simulink subsystem "Diagnostic_Reporter"  (R2023a)
settings: Solver=VariableStepAuto  StartTime=0.0  StopTime=10.0  RelTol=1e-3
undefined symbols (not defined in the file or in its folder): header, key, key_SL_Info, level, message, message_SL_Info, name, name_SL_Info, status, status_SL_Info, value, value_SL_Info, values, values_SL_Info
libraries: ros2lib x13
settings Model: Creator=hollis  LastModifiedBy=john

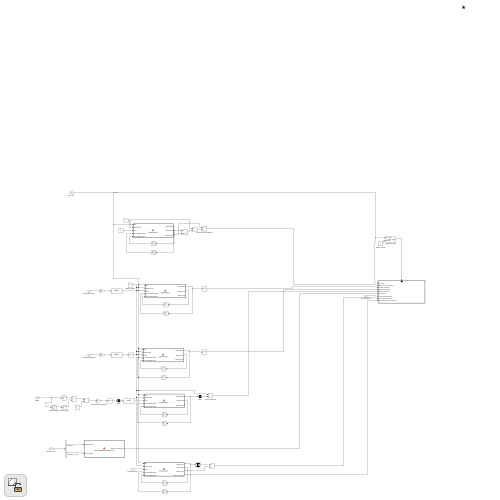
[thumbnail: Simulink's stored preview of the top-level diagram]
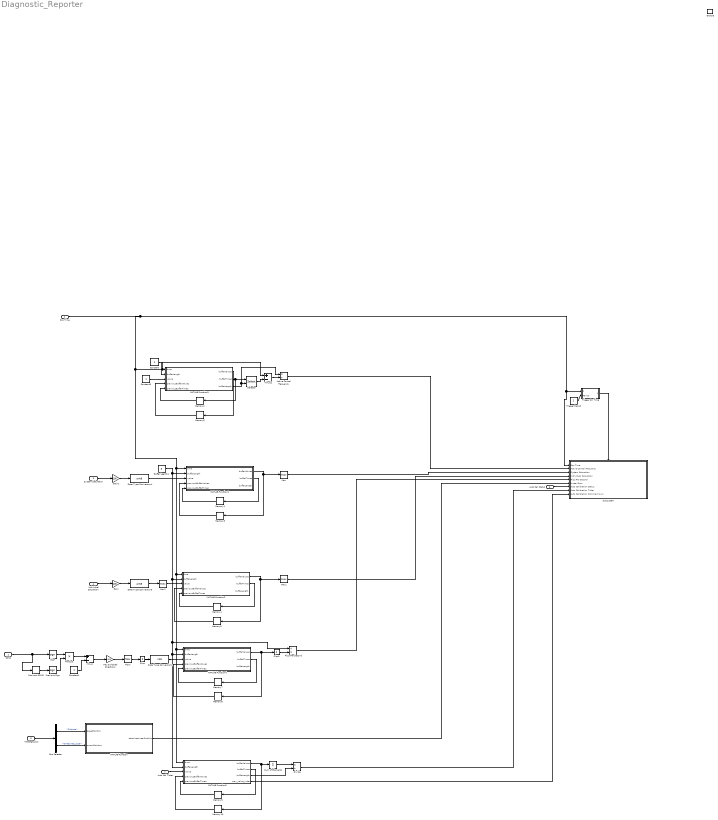
== system Diagnostic_Reporter ==
  Ros Time : Inport
  RPMs : Inport  Port=2
  System Saturation : Inport  Port=3
  Individual Saturation : Inport  Port=4
  message_bus : Inport  Port=5
  Auto Cal Status : Inport  Port=6
  Auto Cal Ticker : Inport  Port=7
  Enable : EnablePort
  Active Control Frequency : Product  Inputs=*/
  Buffer Legnth1 : Constant  Value=3
  Bus Selector : BusSelector  OutputSignals=current_state.DApose,desired_pose.DAdesired_pose
  Constant : Constant
  Constant1 : Constant
  Constant3 : Constant  OutDataTypeStr=single
  Data Type Conversion1 : DataTypeConversion  OutDataTypeStr=int8  SaturateOnIntegerOverflow=off  RndMeth=Floor
  Data Type Conversion3 : DataTypeConversion  OutDataTypeStr=uint8  SaturateOnIntegerOverflow=off  RndMeth=Floor
  Data Type Conversion4 : DataTypeConversion  OutDataTypeStr=uint8  SaturateOnIntegerOverflow=off  RndMeth=Floor
  Divide : Product  Inputs=*/
  Flips : Sum  Inputs=+
  Flips Per Second : Product  Inputs=/*
  Flips1 : Sum  Inputs=+
  Floor : Rounding
  Gain : Gain  Gain=100
  Gain1 : Gain  Gain=100
  Has Switched Directions : Gain  Gain=-1/2
  MATLAB Function : MATLAB Function  TreatAsAtomicUnit=on
  MATLAB Function1 : MATLAB Function  TreatAsAtomicUnit=on
  MATLAB Function2 : MATLAB Function  TreatAsAtomicUnit=on
  MATLAB Function3 : MATLAB Function  TreatAsAtomicUnit=on
  MATLAB Function4 : MATLAB Function  TreatAsAtomicUnit=on
  MATLAB Function5 : MATLAB Function  TreatAsAtomicUnit=on
  Max : MinMax  Function=max
  Max1 : MinMax  Function=max
  Max2 : MinMax  Function=max
  Memory{1..10} (10 alike) : Memory  InitialCondition=[0,0,0,0,0,0,0,0,0,0,0,0,0,0,0,0,0,0,0,0,0,0,0,0,0,0,0,0,0,0,0,0,0,0,0,0,0,0,0,0,0,0,0,0,0,0,0,0,0,0,0,0,0,0,0,0,0,0,0,0,0,0,0,0,0,0,0,0,0,0,0,0,0,0,0,0,0,0,0,0,0,0,0,0,0,0,0,0,0,0,0,0,0,0,0,0,0,0,0,0,0,0,0,0,0,0,0,0,0,0,0,0,0,0,0,0,0,0,0,0,0,0,0,0,0,0,0,0,0,0,0,0,0,0,0,0,0,0,0,0,0,0,0,0,0,0,0,0,0,0,0,0,0,0,0,0,0,0,0,0,0,0,0,0,0,0,0,0,0,0,0,0,0,0,0,0,0,0,0,0,0,0,0,0,0,0,0,0,0,0,0,0,0,0,0,0,0,0,0,0,0,0,0,0,0,0,0,0,0,0,0,0,0,0,0,0,0,0,0,0,0,0,0,0,0,0,0,0,0,0,0,0,0,0,0,0,0,0,0,0,0,0,0,0,0,0,0,0,0,0,0,0,0,0,0,0]
  Minus : Sum  Inputs=+-
  Minus1 : Sum  Inputs=+-
  Previous RPMS : Memory  InitialCondition=[0;0;0;0;0;0;0;0]
  Previous Sign : Signum
  Product : Product
  Selector : Selector  InputPortWidth=256  IndexOptions=Index vector (port)  Indices=[1 3]  OutputSizes=1
  Sign : Signum
  Subsystem : Subsystem
  Sum of Elements : Sum  Inputs=+
  Trigger On Time : Subsystem
  Trigger Period : Constant
  wires:
  MATLAB Function1/1(bufferValues) -> Memory3/1, Max/1
  MATLAB Function2/1(bufferValues) -> Memory5/1, Max1/1
  Gain1/1 -> Data Type Conversion4/1
  Memory3/1 -> MATLAB Function1/4(previousBufferValues)
  MATLAB Function1/2(bufferTimes) -> Memory1/1
  Memory1/1 -> MATLAB Function1/5(previousBufferTimes)
  Memory5/1 -> MATLAB Function2/4(previousBufferValues)
  MATLAB Function2/2(bufferTimes) -> Memory4/1
  Memory4/1 -> MATLAB Function2/5(previousBufferTimes)
  System Saturation/1 -> Gain1/1
  Individual Saturation/1 -> Gain/1
  Gain/1 -> Data Type Conversion3/1
  Data Type Conversion4/1 -> MATLAB Function1/3(value)
  Constant/1 -> MATLAB Function3/2("bufferLength ")
  Constant3/1 -> MATLAB Function3/3(value)
  MATLAB Function3/1(bufferValues) -> Memory6/1
  Memory6/1 -> MATLAB Function3/4(previousBufferValues)
  Memory2/1 -> MATLAB Function3/5(previousBufferTimes)
  MATLAB Function3/2(bufferTimes) -> Selector/1, Memory2/1
  MATLAB Function3/3(bufferLength) -> Selector/2, Active Control Frequency/1
  Selector/1 -> Minus1/2
  Minus1/1 -> Active Control Frequency/2
  Data Type Conversion3/1 -> Max2/1
  Max2/1 -> MATLAB Function2/3(value)
  Active Control Frequency/1 -> Subsystem/2(Active Control Frequency)
  Max/1 -> Subsystem/3(System Saturation)
  Max1/1 -> Subsystem/4(Individual Saturation)
  Trigger Period/1 -> Trigger On Time/2(Period)
  Trigger On Time/1(Trigger Signal) -> Subsystem/Enable
  RPMs/1 -> Sign/1, Previous RPMS/1
  Previous RPMS/1 -> Previous Sign/1
  Sign/1 -> Product/1
  Previous Sign/1 -> Product/2
  Product/1 -> Minus/1
  Constant1/1 -> Minus/2
  Minus/1 -> Has Switched Directions/1
  Has Switched Directions/1 -> Floor/1
  Floor/1 -> Flips/1
  MATLAB Function4/1(bufferValues) -> Memory8/1, Flips1/1
  Memory8/1 -> MATLAB Function4/4(previousBufferValues)
  Memory7/1 -> MATLAB Function4/5(previousBufferTimes)
  MATLAB Function4/2(bufferTimes) -> Memory7/1
  Flips/1 -> Data Type Conversion1/1
  Flips1/1 -> Flips Per Second/2
  Data Type Conversion1/1 -> MATLAB Function4/3(value)
  Flips Per Second/1 -> Subsystem/5(Flips Per Second)
  MATLAB Function/1(absoluteLinearPosition) -> Subsystem/6(Linear Error)
  message_bus/1 -> Bus Selector/1
  Bus Selector/1 -> MATLAB Function/1(targetPosition)  "<DApose>"
  Bus Selector/2 -> MATLAB Function/2(currentPosition)  "<DAdesired_pose>"
  Auto Cal Status/1 -> Subsystem/7(Auto Calibration Status)
  Auto Cal Ticker/1 -> MATLAB Function5/3(value)
  MATLAB Function5/1(bufferValues) -> Memory10/1, Sum of Elements/1
  Memory10/1 -> MATLAB Function5/4(previousBufferValues)
  MATLAB Function5/2(bufferTimes) -> Memory9/1
  Memory9/1 -> MATLAB Function5/5(previousBufferTimes)
  Buffer Legnth1/1 -> MATLAB Function1/2("bufferLength "), MATLAB Function2/2("bufferLength "), MATLAB Function4/2("bufferLength "), MATLAB Function5/2("bufferLength "), Flips Per Second/1
  Ros Time/1 -> Trigger On Time/1(Ros Time), Subsystem/1(Ros Time), MATLAB Function2/1(time), MATLAB Function4/1(time), MATLAB Function5/1(time), MATLAB Function1/1(time), MATLAB Function3/1(time), Minus1/1
  Sum of Elements/1 -> Divide/1
  MATLAB Function5/3(bufferLength) -> Divide/2
  Divide/1 -> Subsystem/8(Auto Calibration Ticker)
  MATLAB Function5/4(max_value_index) -> Subsystem/9(Auto Calibration Dominant Axis)

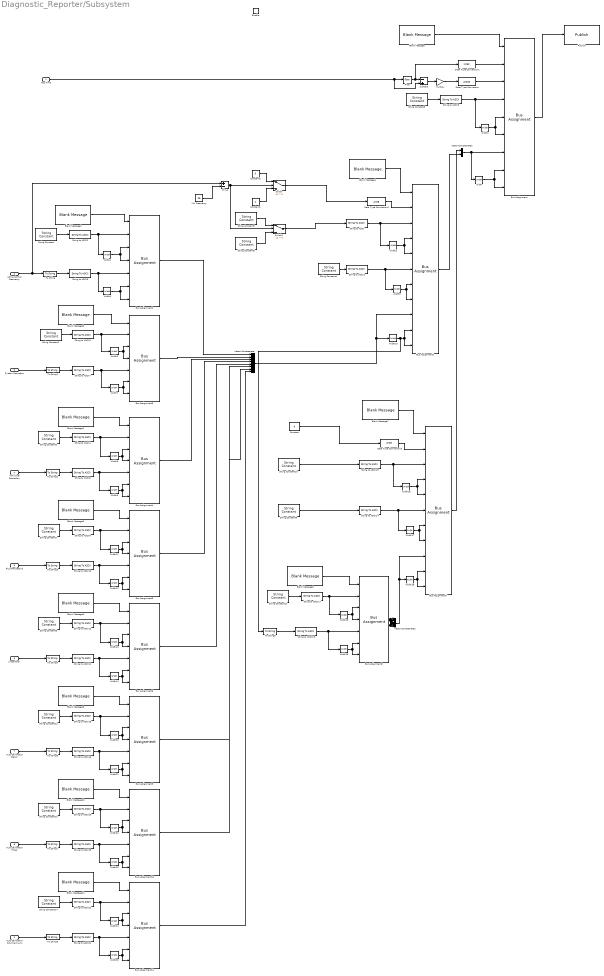
== system Diagnostic_Reporter/Subsystem ==
  Ros Time : Inport
  Active Control Frequency : Inport  Port=2
  System Saturation : Inport  Port=3
  Individual Saturation : Inport  Port=4
  Flips Per Second : Inport  Port=5
  Linear Error : Inport  Port=6
  Auto Calibration Status : Inport  Port=7
  Auto Calibration Ticker : Inport  Port=8
  Auto Calibration Dominant Axis : Inport  Port=9
  Enable : EnablePort
  Blank Message : ros2lib/Blank Message  messageClass=Message  entityType=diagnostic_msgs/DiagnosticArray  messageType=diagnostic_msgs/DiagnosticArray  SampleTime=inf
  Blank Message1 : ros2lib/Blank Message  messageClass=Message  entityType=diagnostic_msgs/DiagnosticStatus  messageType=diagnostic_msgs/DiagnosticStatus  SampleTime=inf
  Blank Message{2..6,8..11} (9 alike) : ros2lib/Blank Message  messageClass=Message  entityType=diagnostic_msgs/KeyValue  messageType=diagnostic_msgs/KeyValue  SampleTime=inf
  Blank Message7 : ros2lib/Blank Message  messageClass=Message  entityType=diagnostic_msgs/DiagnosticStatus  messageType=diagnostic_msgs/DiagnosticStatus  SampleTime=inf
  Bus Assignment : BusAssignment  AssignedSignals=header.stamp.sec,header.stamp.nanosec,header.frame_id,header.frame_id_SL_Info.CurrentLength,header.frame_id_SL_Info.ReceivedLength,status,status_SL_Info.CurrentLength,status_SL_Info.ReceivedLength
  Bus Assignment1 : BusAssignment  AssignedSignals=level,name,name_SL_Info.CurrentLength,name_SL_Info.ReceivedLength,message,message_SL_Info.CurrentLength,message_SL_Info.ReceivedLength,values,values_SL_Info.CurrentLength,values_SL_Info.ReceivedLength
  Bus Assignment{2..6,8..11} (9 alike) : BusAssignment  AssignedSignals=key,key_SL_Info.CurrentLength,key_SL_Info.ReceivedLength,value,value_SL_Info.CurrentLength,value_SL_Info.ReceivedLength
  Bus Assignment7 : BusAssignment  AssignedSignals=level,name,name_SL_Info.CurrentLength,name_SL_Info.ReceivedLength,message,message_SL_Info.CurrentLength,message_SL_Info.ReceivedLength,values,values_SL_Info.CurrentLength,values_SL_Info.ReceivedLength
  Constant : Constant  Value=0
  Constant1 : Constant
  Constant2 : Constant  Value=0
  Data Type Conversion : DataTypeConversion  OutDataTypeStr=uint32  SaturateOnIntegerOverflow=off  RndMeth=Floor
  Data Type Conversion1 : DataTypeConversion  OutDataTypeStr=int32  SaturateOnIntegerOverflow=off  RndMeth=Floor
  Data Type Conversion2 : DataTypeConversion  OutDataTypeStr=uint8  SaturateOnIntegerOverflow=off  RndMeth=Floor
  Data Type Conversion3 : DataTypeConversion  OutDataTypeStr=uint8  SaturateOnIntegerOverflow=off  RndMeth=Floor
  Floor : Rounding
  Min Frequency : Constant  Value=25
  Minus : Sum  Inputs=+-
  Multiply : Gain  Gain=10^9
  Publish : ros2lib/Publish  topicSource=Specify your own  topic=/diagnostics  messageType=diagnostic_msgs/DiagnosticArray  QOSHistory=Keep last  QOSDepth=1  QOSReliability=Reliable  QOSDurability=Volatile
  String Constant : StringConstant  String="\"Active Control Frequency\""
  String Constant1 : StringConstant  String="\"System Limit Saturation\""
  String Constant10 : StringConstant  String="\"Controller Status Values Length\""
  String Constant11 : StringConstant  String="\"Length\""
  String Constant12 : StringConstant  String="\"Auto Tune Status\""
  String Constant13 : StringConstant  String="\"Auto Tune Ticker\""
  String Constant14 : StringConstant  String="\"Auto Tune Dominant Axis\""
  String Constant2 : StringConstant  String="\"Individual Limit Saturation\""
  String Constant3 : StringConstant  String="\"Complete Controller Operating OK\""
  String Constant4 : StringConstant  String="\"System Status is Represented by Frequency and Saturation Values\""
  String Constant5 : StringConstant  String="\"Complete Controller\""
  String Constant6 : StringConstant  String="\"Complete Controller Operating Slow\""
  String Constant7 : StringConstant  String="\"Thruster Direction Flips Frequency\""
  String Constant8 : StringConstant  String="\"Controller Linear Error\""
  String Constant9 : StringConstant  String="\"Length of the Variable Array in System Status\""
  String to ASCII{,1..22} (23 alike) : StringToASCII  OutputVectorSize=128
  Subtract : Sum  Inputs=-+
  Switch : Switch  Criteria=u2 > Threshold  SaturateOnIntegerOverflow=off  InputSameDT=off
  Switch1 : Switch  Criteria=u2 > Threshold  SaturateOnIntegerOverflow=off  InputSameDT=off
  To String{,1..8} (9 alike) : ToString
  Vector Concatenate : Concatenate  NumInputs=8
  Vector Concatenate1 : Concatenate
  Vector Concatenate2 : Concatenate  NumInputs=8
  Width{,1..25} (26 alike) : Width  DataType=uint32
  wires:
  Width25/1 -> Bus Assignment11/7, Bus Assignment11/6
  Auto Calibration Dominant Axis/1 -> To String8/1
  String Constant14/1 -> String to ASCII22/1
  To String8/1 -> String to ASCII21/1
  Width24/1 -> Bus Assignment11/3, Bus Assignment11/4
  Bus Assignment11/1 -> Vector Concatenate/8
  String to ASCII22/1 -> Bus Assignment11/2, Width24/1
  String to ASCII21/1 -> Bus Assignment11/5, Width25/1
  Blank Message11/1 -> Bus Assignment11/1
  String to ASCII20/1 -> Bus Assignment10/2, Width22/1
  Auto Calibration Ticker/1 -> To String7/1
  To String7/1 -> String to ASCII19/1
  String Constant13/1 -> String to ASCII20/1
  Blank Message10/1 -> Bus Assignment10/1
  Width23/1 -> Bus Assignment10/7, Bus Assignment10/6
  Bus Assignment10/1 -> Vector Concatenate/7
  String to ASCII19/1 -> Bus Assignment10/5, Width23/1
  Width22/1 -> Bus Assignment10/3, Bus Assignment10/4
  Bus Assignment9/1 -> Vector Concatenate/6
  String to ASCII18/1 -> Bus Assignment9/2, Width20/1
  To String6/1 -> String to ASCII16/1
  Auto Calibration Status/1 -> To String6/1
  String Constant12/1 -> String to ASCII18/1
  String to ASCII16/1 -> Bus Assignment9/5, Width21/1
  Width20/1 -> Bus Assignment9/3, Bus Assignment9/4
  Blank Message9/1 -> Bus Assignment9/1
  Width21/1 -> Bus Assignment9/7, Bus Assignment9/6
  Bus Assignment8/1 -> Vector Concatenate2/1, Vector Concatenate2/2, Vector Concatenate2/3, Vector Concatenate2/4, Vector Concatenate2/5, Vector Concatenate2/6, Vector Concatenate2/8, Vector Concatenate2/7
  Vector Concatenate2/1 -> Width15/1, Bus Assignment7/9
  Blank Message8/1 -> Bus Assignment8/1
  String to ASCII17/1 -> Bus Assignment8/2, Width18/1
  String Constant11/1 -> String to ASCII17/1
  Width18/1 -> Bus Assignment8/3, Bus Assignment8/4
  String to ASCII15/1 -> Bus Assignment8/5, Width19/1
  Width19/1 -> Bus Assignment8/7, Bus Assignment8/6
  String to ASCII12/1 -> Bus Assignment6/2, Width13/1
  Bus Assignment6/1 -> Vector Concatenate/5
  Width13/1 -> Bus Assignment6/3, Bus Assignment6/4
  Width14/1 -> Bus Assignment6/7, Bus Assignment6/6
  Blank Message6/1 -> Bus Assignment6/1
  String to ASCII11/1 -> Bus Assignment6/5, Width14/1
  Linear Error/1 -> To String4/1
  To String4/1 -> String to ASCII11/1
  String Constant8/1 -> String to ASCII12/1
  Blank Message5/1 -> Bus Assignment5/1
  String to ASCII9/1 -> Bus Assignment5/2, Width11/1
  String Constant7/1 -> String to ASCII9/1
  To String3/1 -> String to ASCII10/1
  Flips Per Second/1 -> To String3/1
  String to ASCII10/1 -> Bus Assignment5/5, Width12/1
  Width11/1 -> Bus Assignment5/3, Bus Assignment5/4
  Bus Assignment5/1 -> Vector Concatenate/4
  Width12/1 -> Bus Assignment5/7, Bus Assignment5/6
  Blank Message4/1 -> Bus Assignment4/1
  String to ASCII7/1 -> Bus Assignment3/5, Width7/1
  Width/1 -> Bus Assignment/9, Bus Assignment/8
  Constant1/1 -> Switch/3
  String to ASCII4/1 -> Bus Assignment4/2, Width8/1
  Subtract/1 -> Multiply/1
  Width9/1 -> Bus Assignment4/7, Bus Assignment4/6
  Bus Assignment/1 -> Publish/1
  To String/1 -> String to ASCII6/1
  Bus Assignment2/1 -> Vector Concatenate/1
  String Constant/1 -> String to ASCII2/1
  Multiply/1 -> Data Type Conversion/1
  Bus Assignment4/1 -> Vector Concatenate/3
  Width5/1 -> Bus Assignment2/6, Bus Assignment2/7
  To String2/1 -> String to ASCII8/1
  Individual Saturation/1 -> To String2/1
  Data Type Conversion/1 -> Bus Assignment/3
  Width4/1 -> Bus Assignment2/3, Bus Assignment2/4
  Ros Time/1 -> Floor/1, Subtract/2
  Minus/1 -> Switch/2, Switch1/2
  System Saturation/1 -> To String1/1
  Width7/1 -> Bus Assignment3/7, Bus Assignment3/6
  Constant2/1 -> Switch/1
  String to ASCII/1 -> Bus Assignment1/3, Width2/1
  Width2/1 -> Bus Assignment1/5, Bus Assignment1/4
  String Constant5/1 -> String to ASCII5/1
  String to ASCII8/1 -> Bus Assignment4/5, Width9/1
  Width1/1 -> Bus Assignment/6, Bus Assignment/5
  Min Frequency/1 -> Minus/2
  Data Type Conversion1/1 -> Bus Assignment/2
  Width6/1 -> Bus Assignment3/4, Bus Assignment3/3
  String Constant6/1 -> Switch1/3
  String Constant3/1 -> Switch1/1
  String to ASCII1/1 -> Bus Assignment1/6, Width3/1
  Data Type Conversion2/1 -> Bus Assignment1/2
  String to ASCII3/1 -> Bus Assignment3/2, Width6/1
  Width3/1 -> Bus Assignment1/7, Bus Assignment1/8
  Width8/1 -> Bus Assignment4/3, Bus Assignment4/4
  Vector Concatenate/1 -> Width10/1, Bus Assignment1/9
  Floor/1 -> Subtract/1, Data Type Conversion1/1
  String to ASCII2/1 -> Bus Assignment2/2, Width4/1
  String Constant1/1 -> String to ASCII3/1
  Vector Concatenate1/1 -> Bus Assignment/7, Width/1
  Blank Message2/1 -> Bus Assignment2/1
  To String1/1 -> String to ASCII7/1
  Active Control Frequency/1 -> To String/1, Minus/1
  Switch/1 -> Data Type Conversion2/1
  String to ASCII5/1 -> Bus Assignment/4, Width1/1
  String Constant2/1 -> String to ASCII4/1
  Switch1/1 -> String to ASCII/1
  Blank Message/1 -> Bus Assignment/1
  Blank Message3/1 -> Bus Assignment3/1
  Blank Message1/1 -> Bus Assignment1/1
  String to ASCII6/1 -> Bus Assignment2/5, Width5/1
  String Constant4/1 -> String to ASCII1/1
  Bus Assignment3/1 -> Vector Concatenate/2
  String to ASCII14/1 -> Bus Assignment7/6, Width17/1
  Data Type Conversion3/1 -> Bus Assignment7/2
  Width15/1 -> Bus Assignment7/10, Bus Assignment7/11
  String to ASCII13/1 -> Bus Assignment7/3, Width16/1
  Width16/1 -> Bus Assignment7/5, Bus Assignment7/4
  Width17/1 -> Bus Assignment7/7, Bus Assignment7/8
  Blank Message7/1 -> Bus Assignment7/1
  Constant/1 -> Data Type Conversion3/1
  String Constant10/1 -> String to ASCII13/1
  Bus Assignment7/1 -> Vector Concatenate1/1
  String Constant9/1 -> String to ASCII14/1
  Bus Assignment1/1 -> Vector Concatenate1/2
  To String5/1 -> String to ASCII15/1
  Width10/1 -> To String5/1, Bus Assignment1/10, Bus Assignment1/11

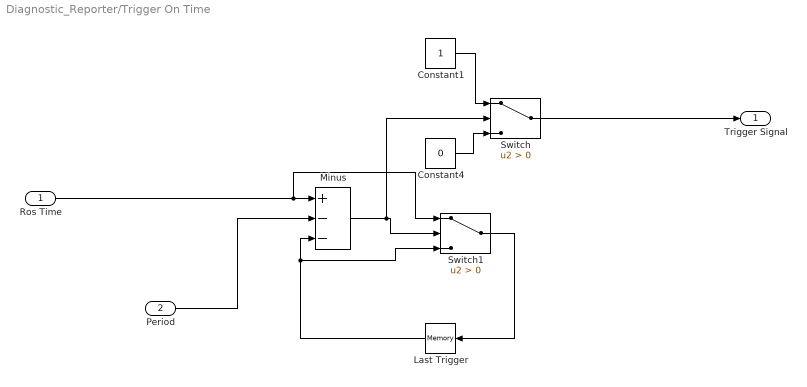
== system Diagnostic_Reporter/Trigger On Time ==
  Ros Time : Inport
  Period : Inport  Port=2
  Constant1 : Constant
  Constant4 : Constant  Value=0
  Last Trigger : Memory
  Minus : Sum  Inputs=+--
  Switch : Switch  Criteria=u2 > Threshold  SaturateOnIntegerOverflow=off  InputSameDT=off
  Switch1 : Switch  Criteria=u2 > Threshold  SaturateOnIntegerOverflow=off  InputSameDT=off
  Trigger Signal : Outport
  wires:
  Period/1 -> Minus/2
  Constant1/1 -> Switch/1
  Minus/1 -> Switch1/2, Switch/2
  Switch1/1 -> Last Trigger/1
  Ros Time/1 -> Minus/1, Switch1/1
  Constant4/1 -> Switch/3
  Last Trigger/1 -> Minus/3, Switch1/3
  Switch/1 -> Trigger Signal/1

== matlab function Diagnostic_Reporter/MATLAB Function1 ==
  data: time input; bufferValues output; bufferLength input; value input; previousBufferValues input; previousBufferTimes input; bufferTimes output; bufferLength output
function [bufferValues, bufferTimes, bufferLength]= bufferValues(time, bufferLength, value, previousBufferValues, previousBufferTimes)

%determine what values to keep in the buffer
%buffer is ordered from newest to oldest
scanning = true;
lastElementToKeep = length(previousBufferTimes) + 1;
lastElementToKeep = min(lastElementToKeep, 256);
while(scanning)
    %increment down
    lastElementToKeep = lastElementToKeep - 1;

    if(lastElementToKeep <= 1 || previousBufferTimes(lastElementToKeep) + bufferLength > time)
        scanning = false;
    end
    
end


bufferValues = zeros(1, 256); 
bufferValues(1) = value;
bufferValues(2:1+lastElementToKeep) = previousBufferValues(1:lastElementToKeep);

bufferTimes = zeros(1, 256);
bufferTimes(1) = time;
bufferTimes(2:1+lastElementToKeep) = previousBufferTimes(1:lastElementToKeep);

bufferLength = (1 + lastElementToKeep);

== matlab function Diagnostic_Reporter/MATLAB Function2 ==
  data: time input; bufferValues output; bufferLength input; value input; previousBufferValues input; previousBufferTimes input; bufferTimes output; bufferLength output
function [bufferValues, bufferTimes, bufferLength]= bufferValues(time, bufferLength, value, previousBufferValues, previousBufferTimes)

%determine what values to keep in the buffer
%buffer is ordered from newest to oldest
scanning = true;
lastElementToKeep = length(previousBufferTimes) + 1;
lastElementToKeep = min(lastElementToKeep, 256);
while(scanning)
    %increment down
    lastElementToKeep = lastElementToKeep - 1;

    if(lastElementToKeep <= 1 || previousBufferTimes(lastElementToKeep) + bufferLength > time)
        scanning = false;
    end
    
end


bufferValues = zeros(1, 256); 
bufferValues(1) = value;
bufferValues(2:1+lastElementToKeep) = previousBufferValues(1:lastElementToKeep);

bufferTimes = zeros(1, 256);
bufferTimes(1) = time;
bufferTimes(2:1+lastElementToKeep) = previousBufferTimes(1:lastElementToKeep);

bufferLength = (1 + lastElementToKeep);

== matlab function Diagnostic_Reporter/MATLAB Function3 ==
  data: time input; bufferValues output; bufferTimes output; bufferLength input; value input; previousBufferValues input; previousBufferTimes input; bufferLength output
function [bufferValues, bufferTimes, bufferLength]= bufferValues(time, bufferLength, value, previousBufferValues, previousBufferTimes)

%determine what values to keep in the buffer
%buffer is ordered from newest to oldest
scanning = true;
lastElementToKeep = length(previousBufferTimes) + 1;
lastElementToKeep = min(lastElementToKeep, 256);
while(scanning)
    %increment down
    lastElementToKeep = lastElementToKeep - 1;

    if(lastElementToKeep <= 1 || previousBufferTimes(lastElementToKeep) + bufferLength > time)
        scanning = false;
    end
    
end


bufferValues = zeros(1, 256); 
bufferValues(1) = value;
bufferValues(2:1+lastElementToKeep) = previousBufferValues(1:lastElementToKeep);

bufferTimes = zeros(1, 256);
bufferTimes(1) = time;
bufferTimes(2:1+lastElementToKeep) = previousBufferTimes(1:lastElementToKeep);

bufferLength = (1 + lastElementToKeep);

== matlab function Diagnostic_Reporter/MATLAB Function4 ==
  data: time input; bufferValues output; bufferLength input; value input; previousBufferValues input; previousBufferTimes input; bufferTimes output; bufferLength output
function [bufferValues, bufferTimes, bufferLength]= bufferValues(time, bufferLength, value, previousBufferValues, previousBufferTimes)

%determine what values to keep in the buffer
%buffer is ordered from newest to oldest
scanning = true;
lastElementToKeep = length(previousBufferTimes) + 1;
lastElementToKeep = min(lastElementToKeep, 256);
while(scanning)
    %increment down
    lastElementToKeep = lastElementToKeep - 1;

    if(lastElementToKeep <= 1 || previousBufferTimes(lastElementToKeep) + bufferLength > time)
        scanning = false;
    end
    
end


bufferValues = zeros(1, 256); 
bufferValues(1) = value;
bufferValues(2:1+lastElementToKeep) = previousBufferValues(1:lastElementToKeep);

bufferTimes = zeros(1, 256);
bufferTimes(1) = time;
bufferTimes(2:1+lastElementToKeep) = previousBufferTimes(1:lastElementToKeep);

bufferLength = (1 + lastElementToKeep);

== matlab function Diagnostic_Reporter/MATLAB Function ==
  data: targetPosition input; absoluteLinearPosition output; currentPosition input
function absoluteLinearPosition = convertToAbsoluteDistancce(targetPosition, currentPosition)

absoluteLinearPosition = sqrt((targetPosition(1) - currentPosition(1))^2 + (targetPosition(2) - currentPosition(2))^2 + (targetPosition(3) - currentPosition(3))^2);

== matlab function Diagnostic_Reporter/MATLAB Function5 ==
  data: time input; bufferValues output; bufferLength input; value input; previousBufferValues input; previousBufferTimes input; bufferTimes output; bufferLength output; max_value_index output
function [bufferValues, bufferTimes, bufferLength, max_value_index]= bufferValues(time, bufferLength, value, previousBufferValues, previousBufferTimes)

%find the dominant axis - it is understood that this is incorrect when
%the buffer is taken into consideration, however, it likely not worth being
%perfect...
max_value = 0;
max_value_index = -1;
for index=1:6
    if(abs(max_value) < abs(value(index)))
        max_value = value(index);
        max_value_index = index;
    end
end

%determine what values to keep in the buffer
%buffer is ordered from newest to oldest
scanning = true;
lastElementToKeep = length(previousBufferTimes) + 1;
lastElementToKeep = min(lastElementToKeep, 256);
while(scanning)
    %increment down
    lastElementToKeep = lastElementToKeep - 1;

    if(lastElementToKeep <= 1 || previousBufferTimes(lastElementToKeep) + bufferLength > time)
        scanning = false;
    end
    
end


bufferValues = zeros(1, 256); 
bufferValues(1) = max_value;
bufferValues(2:1+lastElementToKeep) = previousBufferValues(1:lastElementToKeep);

bufferTimes = zeros(1, 256);
bufferTimes(1) = time;
bufferTimes(2:1+lastElementToKeep) = previousBufferTimes(1:lastElementToKeep);

bufferLength = (1 + lastElementToKeep);
